simulink model "Mdl_DLR"  (R2021b)
settings: Solver=FixedStepAuto  StartTime=0.0  StopTime=10.0  FixedStep=DT_s  RelTol=1e-3
values from neighbouring files (symbols this model uses):
  BEMTPitchMax_deg = -30.0    [DD_Mdl.sldd]    (also in initRotorsimulationNREL5MW.m = -30)
  BladeLength_m = 61.5    [DD_Mdl.sldd]    (also in initRotorsimulationNREL5MW.m)
  BladeMass_kg = 17740.0    [DD_Mdl.sldd]    (also in initRotorsimulationNREL5MW.m = 17740)
  BladePitchMax_deg = 0.0    [DD_Mdl.sldd]    (also in initRotorsimulationNREL5MW.m = 0)
  BladePitchrateNorm_degpers = 3.0    [DD_Mdl.sldd]    (also in initRotorsimulationNREL5MW.m = 3)
  BladePitchrateStop_degpers = 9.0    [DD_Mdl.sldd]    (also in initRotorsimulationNREL5MW.m = 9)
  BladePitchStart_deg = -85.0    [DD_Mdl.sldd]    (also in initRotorsimulationNREL5MW.m = -85)
  BladePrecone_deg = 2.5    [DD_Mdl.sldd]    (also in initRotorsimulationNREL5MW.m)
  BladeTwist_deg = 13.308 13.308 13.308 13.308 13.308 13.308 13.308 13.308 13.308 13.308 13.308 13.308 13.181 12.848 12.192 11.561 11.072 10.792 10.232 9.672 9.11 8.534 7.932 7.321 6.711 6.122 5.546 4.971 4.401 3.834 3.332 2.89 2.503 2.116 1.73 1.342 0.954 0.76 0.574 0.404 0.319 0.253 0.216 0.178 0.14 0.101 0.062 0.023 0.0    [DD_Mdl.sldd]    (also in initRotorsimulationNREL5MW.m = [13.308 13.308 13.308 13.308 13.308 13.308 13.308 13.308 13.)
  cperR = 0.054 0.054 0.056 0.058 0.06 0.061 0.063 0.065 0.067 0.069 0.07 0.072 0.073 0.073 0.073 0.074 0.073 0.072 0.071 0.069 0.068 0.066 0.064 0.062 0.06 0.058 0.056 0.054 0.052 0.05 0.049 0.047 0.045 0.043 0.041 0.039 0.037 0.036 0.035 0.033 0.032 0.03 0.028 0.026 0.024 0.022 0.02 0.018 0.017    [DD_Mdl.sldd]    (also in initRotorsimulationNREL5MW.m = [0.054 0.054 0.056 0.058 0.060 0.061 0.063 0.065 0.067 0.069)
  Cut_OffWindSpeed_mpers = 25.0    [DD_Mdl.sldd]    (also in initRotorsimulationNREL5MW.m = 25)
  DownwashCorrection = 0.26    [DD_Mdl.sldd]    (also in initRotorsimulationNREL5MW.m)
  DownwashModelSwitch = 3.0    [DD_Mdl.sldd]    (also in initRotorsimulationNREL5MW.m = 3)
  drperR = 0.024 0.003 0.016 0.016 0.016 0.016 0.016 0.016 0.016 0.016 0.016 0.016 0.016 0.016 0.016 0.016 0.016 0.016 0.032 0.032 0.032 0.032 0.032 0.032 0.032 0.032 0.032 0.032 0.032 0.032 0.032 0.032 0.032 0.032 0.032 0.032 0.032 0.016 0.016 0.016 0.008 0.008 0.008 0.008 0.008 0.008 0.008 0.008 0.005    [DD_Mdl.sldd]    (also in initRotorsimulationNREL5MW.m = [0.024 0.003 0.016 0.016 0.016 0.016 0.016 0.016 0.016 0.016)
  DT = 0.008    [DD_LPV.sldd]    (also in DD_Mdl.sldd)
  DT_s = 0.008    [DD_Mdl.sldd]    (also in initRotorsimulationNREL5MW.m = 0.01)
  g_mpers_2 = 9.81    [DD_Mdl.sldd]    (also in initRotorsimulationNREL5MW.m)
  GeneratorEfficiency = 0.944    [DD_Mdl.sldd]    (also in initRotorsimulationNREL5MW.m)
  GeneratorOptimalModeGain_Nmper_radpers2 = 2128600    [initRotorsimulationNREL5MW.m]
  HubRadius_m = 1.5    [DD_Mdl.sldd]    (also in initRotorsimulationNREL5MW.m)
  Ki = 0.3    [initRotorsimulationNREL5MW.m]
  Kp = 0.1    [initRotorsimulationNREL5MW.m]
  mpermBl = 0.058 0.008 0.044 0.043 0.042 0.034 0.026 0.024 0.023 0.022 0.023 0.024 0.024 0.023 0.022 0.02 0.02 0.02 0.039 0.038 0.037 0.036 0.034 0.033 0.03 0.029 0.028 0.025 0.023 0.021 0.019 0.018 0.016 0.015 0.012 0.011 0.01 0.005 0.004 0.004 0.002 0.002 0.002 0.002 0.001 0.001 0.001 0.0 0.0    [DD_Mdl.sldd]    (also in initRotorsimulationNREL5MW.m = [0.058 0.008 0.044 0.043 0.042 0.034 0.026 0.024 0.023 0.022)
  nBl = 3.0    [DD_Mdl.sldd]    (also in initRotorsimulationNREL5MW.m = 3)
  nR = 49.0    [DD_Mdl.sldd]    (also in initRotorsimulationNREL5MW.m = length(drperR))
  Overhang_m = 5.0    [DD_Mdl.sldd]    (also in initRotorsimulationNREL5MW.m = 5)
  RatedOmega_RPM = 12.1    [DD_Mdl.sldd]    (also in initRotorsimulationNREL5MW.m)
  RatedWindSpeed_mpers = 11.4    [DD_Mdl.sldd]    (also in initRotorsimulationNREL5MW.m)
  rho_kgperm3 = 1.225    [DD_Mdl.sldd]    (also in initRotorsimulationNREL5MW.m)
  rperR = 0.024 0.027 0.043 0.059 0.075 0.09 0.106 0.122 0.138 0.154 0.17 0.186 0.202 0.217 0.233 0.249 0.265 0.281 0.313 0.344 0.376 0.408 0.44 0.471 0.503 0.535 0.567 0.598 0.63 0.662 0.694 0.725 0.757 0.789 0.821 0.852 0.884 0.9 0.916 0.932 0.94 0.948 0.956 0.963 0.971 0.979 0.987 0.995 1.0    [DD_Mdl.sldd]    (also in initRotorsimulationNREL5MW.m = [0.024 0.027 0.043 0.059 0.075 0.090 0.106 0.122 0.138 0.154)
  Shafttilt_deg = 5.0    [DD_Mdl.sldd]    (also in initRotorsimulationNREL5MW.m = 5)
  TipSpeedLoss = 0.0    [DD_Mdl.sldd]    (also in initRotorsimulationNREL5MW.m = 0)
  TowerDamOnperoff = 0.0    [DD_Mdl.sldd]    (also in initRotorsimulationNREL5MW.m = 0)
  TowerDragCoefficient = 0.35    [DD_Mdl.sldd]    (also in initRotorsimulationNREL5MW.m)
  TowerRadius_m = 1.935    [DD_Mdl.sldd]    (also in initRotorsimulationNREL5MW.m)
  wecs = 3.0    [DD_Mdl.sldd]    (also in DD_Mdl1.sldd = 3.0
libraries: simulink x3
(part 2 of 2)

== system Mdl_DLR/WEA-Anlage/Blattaerodynamik/Tip&Hub-Loss-Faktor ==
  sin phi : Inport
  Divide : Product  Inputs=*/
  Divide1 : Product  Inputs=*/
  Divide2 : Product  Inputs=*/
  Fhub : Scope
  Ftip : Scope
  Gain : Gain  Gain=1/2
  Gain1 : Gain  Gain=-1
  Gain2 : Gain  Gain=2/pi
  Gain3 : Gain  Gain=-1
  Gain4 : Gain  Gain=2/pi
  Math Function : Math  SignedPower=on  SaturateOnIntegerOverflow=on
  Math Function1 : Math  SignedPower=on  SaturateOnIntegerOverflow=on
  Mux : Mux  Inputs=3
  Mux1 : Mux  Inputs=3
  Product : Product  RndMeth=Zero
  Product1 : Product  RndMeth=Zero
  Product2 : Product  RndMeth=Zero
  Saturation : Saturate  UpperLimit=10  LowerLimit=0.01
  Saturation1 : Saturate  UpperLimit=inf  LowerLimit=0
  Sum : Sum  Inputs=|+-
  Sum1 : Sum  Inputs=|+-
  Trigonometric Function : Trigonometry  Operator=acos
  Trigonometric Function1 : Trigonometry  Operator=acos
  F : Outport  VectorParamsAs1DForOutWhenUnconnected=off
  wires:
  [R] -> Sum/1
  [nBl] -> Gain/1
  Sum/1 -> Divide1/1
  Math Function/1 -> Trigonometric Function/1
  Gain1/1 -> Math Function/1
  sin phi/1 -> Saturation/1
  [r_eff] -> Sum/2, Divide1/2, Sum1/1
  Math Function1/1 -> Trigonometric Function1/1
  Gain3/1 -> Math Function1/1
  Product/1 -> F/1  "F"
  Gain/1 -> Divide/1
  Saturation/1 -> Divide/2
  Sum1/1 -> Divide2/1
  [R_hub] -> Divide2/2, Sum1/2
  Divide/1 -> Product1/1, Product2/1
  Product1/1 -> Gain1/1
  Product2/1 -> Saturation1/1
  Trigonometric Function/1 -> Gain4/1
  Trigonometric Function1/1 -> Gain2/1
  Gain4/1 -> Product/1, Ftip/1  "Ftip"
  Gain2/1 -> Product/2, Fhub/1  "Fhub"
  Saturation1/1 -> Gain3/1
  Divide1/1 -> Mux/1, Mux/2, Mux/3
  Mux/1 -> Product1/2
  Divide2/1 -> Mux1/1, Mux1/2, Mux1/3
  Mux1/1 -> Product2/2

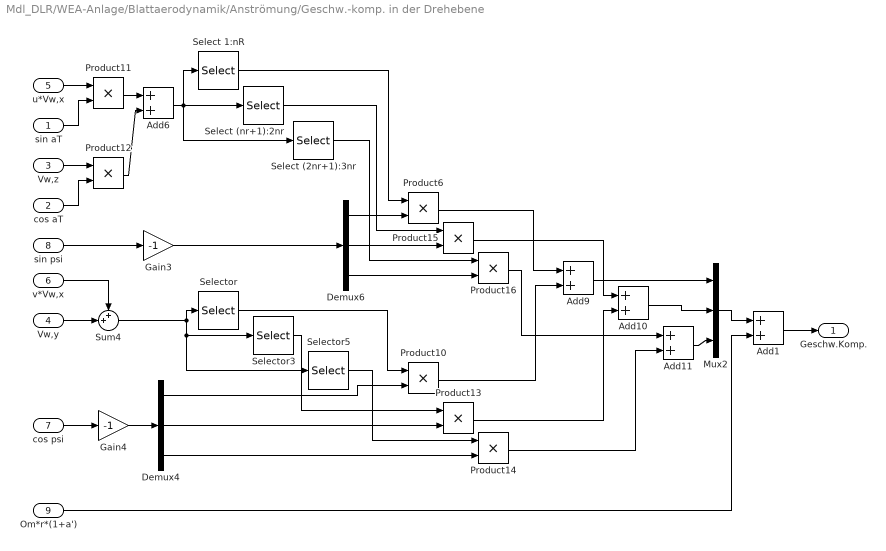
== system Mdl_DLR/WEA-Anlage/Blattaerodynamik/Anströmung/Geschw.-komp. in der Drehebene ==
  sin aT : Inport
  cos aT : Inport  Port=2
  Vw,z : Inport  Port=3
  Vw,y : Inport  Port=4
  u*Vw,x : Inport  Port=5
  v*Vw,x : Inport  Port=6
  cos psi : Inport  Port=7
  sin psi : Inport  Port=8
  Om*r*(1+a') : Inport  Port=9
  Add{1,6,9..11} (5 alike) : Sum
  Demux4 : Demux  Outputs=3
  Demux6 : Demux  Outputs=3
  Gain3 : Gain  Gain=-1
  Gain4 : Gain  Gain=-1
  Mux2 : Mux  Inputs=3
  Product{6,10..16} (8 alike) : Product  RndMeth=Zero
  Select (2nr+1):3nr : Selector  InputPortWidth=3*nR  IndexOptions=Index vector (dialog)  Indices=[2*nR+1:3*nR]  OutputSizes=1
  Select (nr+1):2nr : Selector  InputPortWidth=3*nR  IndexOptions=Index vector (dialog)  Indices=[nR+1:2*nR]  OutputSizes=1
  Select 1:nR : Selector  InputPortWidth=3*nR  IndexOptions=Index vector (dialog)  Indices=[1:nR]  OutputSizes=1
  Selector : Selector  InputPortWidth=3*nR  IndexOptions=Index vector (dialog)  Indices=[1:nR]  OutputSizes=1
  Selector3 : Selector  InputPortWidth=3*nR  IndexOptions=Index vector (dialog)  Indices=[nR+1:2*nR]  OutputSizes=1
  Selector5 : Selector  InputPortWidth=3*nR  IndexOptions=Index vector (dialog)  Indices=[2*nR+1:3*nR]  OutputSizes=1
  Sum4 : Sum  Inputs=++|
  Geschw.Komp. : Outport  VectorParamsAs1DForOutWhenUnconnected=off
  wires:
  Demux6/1 -> Product6/2
  Demux6/2 -> Product15/2
  Product6/1 -> Add9/1
  Product15/1 -> Add10/1
  Select 1:nR/1 -> Product6/1
  Product13/1 -> Add10/2
  Product16/1 -> Add11/1
  Add6/1 -> Select (nr+1):2nr/1, Select 1:nR/1, Select (2nr+1):3nr/1
  Demux6/3 -> Product16/2
  Product14/1 -> Add11/2
  Selector5/1 -> Product14/1
  Selector/1 -> Product10/1
  Product10/1 -> Add9/2
  Demux4/3 -> Product14/2
  Demux4/2 -> Product13/2
  Demux4/1 -> Product10/2
  Product12/1 -> Add6/2
  Product11/1 -> Add6/1
  Gain4/1 -> Demux4/1
  Add11/1 -> Mux2/3
  Add10/1 -> Mux2/2
  Add9/1 -> Mux2/1
  Gain3/1 -> Demux6/1
  u*Vw,x/1 -> Product11/1
  sin aT/1 -> Product11/2
  Vw,z/1 -> Product12/1
  cos aT/1 -> Product12/2
  cos psi/1 -> Gain4/1
  sin psi/1 -> Gain3/1
  v*Vw,x/1 -> Sum4/1
  Vw,y/1 -> Sum4/2
  Sum4/1 -> Selector5/1, Selector3/1, Selector/1
  Select (nr+1):2nr/1 -> Product15/1
  Selector3/1 -> Product13/1
  Select (2nr+1):3nr/1 -> Product16/1
  Mux2/1 -> Add1/1
  Add1/1 -> Geschw.Komp./1
  Om*r*(1+a')/1 -> Add1/2

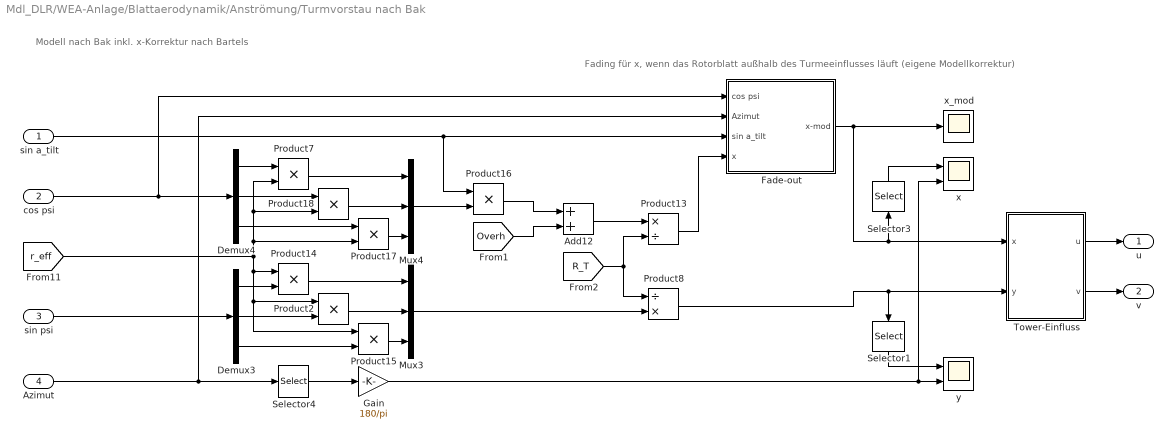
== system Mdl_DLR/WEA-Anlage/Blattaerodynamik/Anströmung/Turmvorstau nach Bak ==
  note: Fading für x, wenn das Rotorblatt außhalb des Turmeeinflusses läuft (eigene Modellkorrektur)
  note: Modell nach Bak inkl. x-Korrektur nach Bartels
  sin a_tilt : Inport
  cos psi : Inport  Port=2
  sin psi : Inport  Port=3
  Azimut : Inport  Port=4
  " x_mod " : Scope
  Add12 : Sum
  Demux3 : Demux  Outputs=3
  Demux4 : Demux  Outputs=3
  Fade-out : Subsystem
  Gain : Gain  Gain=180/pi
  Mux3 : Mux  Inputs=3
  Mux4 : Mux  Inputs=3
  Product13 : Product  Inputs=*/  RndMeth=Zero
  Product{2,7,14..18} (7 alike) : Product  RndMeth=Zero
  Product8 : Product  Inputs=/*  RndMeth=Zero
  Selector1 : Selector  InputPortWidth=3*nR  IndexOptions=Index vector (dialog)  Indices=[1:nR]  OutputSizes=1
  Selector3 : Selector  InputPortWidth=3*nR  IndexOptions=Index vector (dialog)  Indices=[1:nR]  OutputSizes=1
  Selector4 : Selector  InputPortWidth=3  IndexOptions=Index vector (dialog)  Indices=[1]  OutputSizes=1
  Tower-Einfluss : Subsystem
  x : Scope  NumInputPorts=2
  y : Scope  NumInputPorts=2
  u : Outport  VectorParamsAs1DForOutWhenUnconnected=off
  v : Outport  Port=2  VectorParamsAs1DForOutWhenUnconnected=off
  wires:
  Product8/1 -> Tower-Einfluss/2(y), Selector1/1
  [Overh] -> Add12/2
  Add12/1 -> Product13/1
  [R_T] -> Product13/2, Product8/1
  Mux3/1 -> Product8/2
  Product15/1 -> Mux3/3
  Product2/1 -> Mux3/2
  Product14/1 -> Mux3/1
  Demux3/1 -> Product14/2
  Demux3/2 -> Product2/2
  Demux3/3 -> Product15/2
  Product17/1 -> Mux4/3
  Product18/1 -> Mux4/2
  Product7/1 -> Mux4/1
  Demux4/1 -> Product7/1
  Demux4/2 -> Product18/1
  Demux4/3 -> Product17/1
  Selector1/1 -> y/1
  Selector3/1 -> x/1
  Selector4/1 -> Gain/1
  Tower-Einfluss/1(u) -> u/1
  Tower-Einfluss/2(v) -> v/1
  [r_eff] -> Product14/1, Product2/1, Product15/1, Product17/2, Product18/2, Product7/2
  sin psi/1 -> Demux3/1
  Azimut/1 -> Selector4/1, Fade-out/2(Azimut)
  cos psi/1 -> Demux4/1, Fade-out/1(cos psi)
  Gain/1 -> y/2, x/2
  Mux4/1 -> Product16/2
  sin a_tilt/1 -> Product16/1, Fade-out/3(sin a_tilt)
  Product16/1 -> Add12/1
  Product13/1 -> Fade-out/4(x)
  Fade-out/1(" x-mod") -> " x_mod "/1, Tower-Einfluss/1(x), Selector3/1

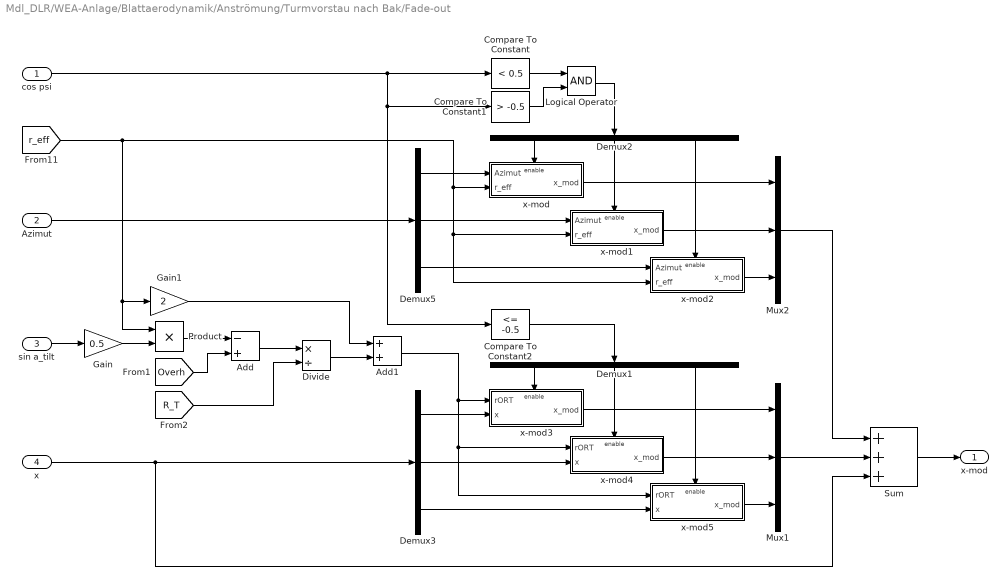
== system Mdl_DLR/WEA-Anlage/Blattaerodynamik/Anströmung/Turmvorstau nach Bak/Fade-out ==
  cos psi : Inport
  Azimut : Inport  Port=2
  sin a_tilt : Inport  Port=3
  x : Inport  Port=4
  Add : Sum  Inputs=-+
  Add1 : Sum
  Compare To Constant : simulink/Logic and Bit Operations/Compare To Constant  relop=<  const=0.5  OutDataTypeStr=boolean  ZeroCross=off
  Compare To Constant1 : simulink/Logic and Bit Operations/Compare To Constant  relop=>  const=-0.5  OutDataTypeStr=boolean  ZeroCross=off
  Compare To Constant2 : simulink/Logic and Bit Operations/Compare To Constant  relop=<=  const=-0.5  OutDataTypeStr=boolean  ZeroCross=off
  Demux{1..3,5} (4 alike) : Demux  Outputs=3
  Divide : Product  Inputs=*/
  Gain : Gain  Gain=0.5
  Gain1 : Gain  Gain=2
  Logical Operator : Logic  AllPortsSameDT=off  OutDataTypeStr=boolean
  Mux1 : Mux  Inputs=3
  Mux2 : Mux  Inputs=3
  Product : Product  RndMeth=Zero
  Sum : Sum  Inputs=+++
  x-mod : Subsystem  TreatAsAtomicUnit=on
  x-mod1 : Subsystem  TreatAsAtomicUnit=on
  x-mod2 : Subsystem  TreatAsAtomicUnit=on
  x-mod3 : Subsystem  TreatAsAtomicUnit=on
  x-mod4 : Subsystem  TreatAsAtomicUnit=on
  x-mod5 : Subsystem  TreatAsAtomicUnit=on
  " x-mod" : Outport  VectorParamsAs1DForOutWhenUnconnected=off
  wires:
  x-mod2/1(x_mod) -> Mux2/3
  Demux2/1 -> x-mod/Enable
  x-mod1/1(x_mod) -> Mux2/2
  Demux5/3 -> x-mod2/1(Azimut)
  Demux5/2 -> x-mod1/1(Azimut)
  Demux5/1 -> x-mod/1(Azimut)
  Demux2/2 -> x-mod1/Enable
  Demux2/3 -> x-mod2/Enable
  cos psi/1 -> Compare To Constant/1, Compare To Constant1/1, Compare To Constant2/1
  Azimut/1 -> Demux5/1
  Compare To Constant/1 -> Logical Operator/1
  Compare To Constant1/1 -> Logical Operator/2
  Logical Operator/1 -> Demux2/1
  Sum/1 -> " x-mod"/1
  Compare To Constant2/1 -> Demux1/1
  Demux1/1 -> x-mod3/Enable
  Demux3/1 -> x-mod3/2(x)
  x/1 -> Demux3/1, Sum/3
  x-mod3/1(x_mod) -> Mux1/1
  Demux1/3 -> x-mod5/Enable
  x-mod5/1(x_mod) -> Mux1/3
  x-mod4/1(x_mod) -> Mux1/2
  Demux3/2 -> x-mod4/2(x)
  Demux3/3 -> x-mod5/2(x)
  Demux1/2 -> x-mod4/Enable
  x-mod/1(x_mod) -> Mux2/1
  [r_eff] -> x-mod/2(r_eff), x-mod1/2(r_eff), x-mod2/2(r_eff), Product/1, Gain1/1
  Mux2/1 -> Sum/1
  Mux1/1 -> Sum/2
  sin a_tilt/1 -> Gain/1
  Gain/1 -> Product/2
  Product/1 -> Add/1
  [Overh] -> Add/2
  Add/1 -> Divide/1
  [R_T] -> Divide/2
  Divide/1 -> Add1/2
  Gain1/1 -> Add1/1
  Add1/1 -> x-mod3/1(rORT), x-mod4/1(rORT), x-mod5/1(rORT)

== system Mdl_DLR/WEA-Anlage/Blattaerodynamik/Anströmung/Turmvorstau nach Bak/Tower-Einfluss ==
  x : Inport
  y : Inport  Port=2
  Add12 : Sum  Inputs=+-+
  Add13 : Sum
  Constant1 : Constant
  Constant4 : Constant  Value=0.1
  Gain6 : Gain  Gain=1/(2*pi)
  Gain7 : Gain  Gain=2
  Math Function2 : Math  Operator=square  SignedPower=on  SaturateOnIntegerOverflow=on
  Math Function3 : Math  Operator=square  SignedPower=on  SaturateOnIntegerOverflow=on
  Math Function5 : Math  Operator=square  SignedPower=on  SaturateOnIntegerOverflow=on
  Product13 : Product  Inputs=/*  RndMeth=Zero
  Product14 : Product  Inputs=/**  RndMeth=Zero
  Product2 : Product  Inputs=*/  RndMeth=Zero
  Product7 : Product  Inputs=/**  RndMeth=Zero
  Product8 : Product  RndMeth=Zero
  Sum4 : Sum  Inputs=++|
  Sum5 : Sum  Inputs=|+-
  Sum6 : Sum  Inputs=++|
  u : Outport  VectorParamsAs1DForOutWhenUnconnected=off
  v : Outport  Port=2  VectorParamsAs1DForOutWhenUnconnected=off
  wires:
  Constant1/1 -> Add12/1
  Constant4/1 -> Sum4/1
  Sum4/1 -> Math Function2/1, Product7/2, Product8/1
  y/1 -> Product14/3, Product8/2, Math Function3/1
  Math Function2/1 -> Sum5/1, Sum6/1
  Math Function3/1 -> Sum5/2, Sum6/2
  Sum5/1 -> Product2/1
  Sum6/1 -> Math Function5/1, Product7/1, Product14/1
  Product2/1 -> Add12/2
  [cd_T] -> Gain6/1
  Gain6/1 -> Product7/3, Product14/2
  Product7/1 -> Add12/3
  Math Function5/1 -> Product2/2, Product13/1
  Product8/1 -> Gain7/1
  Gain7/1 -> Product13/2
  Product13/1 -> Add13/1
  Product14/1 -> Add13/2
  x/1 -> Sum4/2
  Add12/1 -> u/1  "u"
  Add13/1 -> v/1  "v"

== system Mdl_DLR/WEA-Anlage/Blattaerodynamik/Anströmung/Turmvorstau nach Bak/Fade-out/x-mod ==
  Azimut : Inport
  r_eff : Inport  Port=2
  Enable : EnablePort  StatesWhenEnabling=reset
  Add1 : Sum
  Constant3 : Constant
  Gain1 : Gain  Gain=3
  Product4 : Product  RndMeth=Zero
  Trigonometric Function6 : Trigonometry  Operator=cos
  x_mod : Outport  OutputWhenDisabled=reset  InitialOutput=0  VectorParamsAs1DForOutWhenUnconnected=off
  wires:
  Constant3/1 -> Add1/1
  Gain1/1 -> Trigonometric Function6/1
  Trigonometric Function6/1 -> Add1/2
  Add1/1 -> Product4/1
  Product4/1 -> x_mod/1
  Azimut/1 -> Gain1/1
  r_eff/1 -> Product4/2

== system Mdl_DLR/WEA-Anlage/Blattaerodynamik/Anströmung/Turmvorstau nach Bak/Fade-out/x-mod1 ==
  Azimut : Inport
  r_eff : Inport  Port=2
  Enable : EnablePort  StatesWhenEnabling=reset
  Add1 : Sum
  Constant3 : Constant
  Gain1 : Gain  Gain=3
  Product4 : Product  RndMeth=Zero
  Trigonometric Function6 : Trigonometry  Operator=cos
  x_mod : Outport  OutputWhenDisabled=reset  InitialOutput=0  VectorParamsAs1DForOutWhenUnconnected=off
  wires:
  r_eff/1 -> Product4/2
  Azimut/1 -> Gain1/1
  Product4/1 -> x_mod/1
  Add1/1 -> Product4/1
  Trigonometric Function6/1 -> Add1/2
  Gain1/1 -> Trigonometric Function6/1
  Constant3/1 -> Add1/1

== system Mdl_DLR/WEA-Anlage/Blattaerodynamik/Anströmung/Turmvorstau nach Bak/Fade-out/x-mod2 ==
  Azimut : Inport
  r_eff : Inport  Port=2
  Enable : EnablePort  StatesWhenEnabling=reset
  Add1 : Sum
  Constant3 : Constant
  Gain1 : Gain  Gain=3
  Product4 : Product  RndMeth=Zero
  Trigonometric Function6 : Trigonometry  Operator=cos
  x_mod : Outport  OutputWhenDisabled=reset  InitialOutput=0  VectorParamsAs1DForOutWhenUnconnected=off
  wires:
  Constant3/1 -> Add1/1
  Gain1/1 -> Trigonometric Function6/1
  Trigonometric Function6/1 -> Add1/2
  Add1/1 -> Product4/1
  Product4/1 -> x_mod/1
  Azimut/1 -> Gain1/1
  r_eff/1 -> Product4/2

== system Mdl_DLR/WEA-Anlage/Blattaerodynamik/Anströmung/Turmvorstau nach Bak/Fade-out/x-mod3 ==
  rORT : Inport
  x : Inport  Port=2
  Enable : EnablePort  StatesWhenEnabling=reset
  Sum : Sum  Inputs=|+-
  x_mod : Outport  OutputWhenDisabled=reset  InitialOutput=0  VectorParamsAs1DForOutWhenUnconnected=off
  wires:
  rORT/1 -> Sum/1
  x/1 -> Sum/2
  Sum/1 -> x_mod/1

== system Mdl_DLR/WEA-Anlage/Blattaerodynamik/Anströmung/Turmvorstau nach Bak/Fade-out/x-mod4 ==
  rORT : Inport
  x : Inport  Port=2
  Enable : EnablePort  StatesWhenEnabling=reset
  Sum : Sum  Inputs=|+-
  x_mod : Outport  OutputWhenDisabled=reset  InitialOutput=0  VectorParamsAs1DForOutWhenUnconnected=off
  wires:
  Sum/1 -> x_mod/1
  x/1 -> Sum/2
  rORT/1 -> Sum/1

== system Mdl_DLR/WEA-Anlage/Blattaerodynamik/Anströmung/Turmvorstau nach Bak/Fade-out/x-mod5 ==
  rORT : Inport
  x : Inport  Port=2
  Enable : EnablePort  StatesWhenEnabling=reset
  Sum : Sum  Inputs=|+-
  x_mod : Outport  OutputWhenDisabled=reset  InitialOutput=0  VectorParamsAs1DForOutWhenUnconnected=off
  wires:
  rORT/1 -> Sum/1
  x/1 -> Sum/2
  Sum/1 -> x_mod/1
